simulink model "untitled"  (R2022a)
settings: Solver=FixedStepDiscrete  StartTime=0.0  StopTime=10.0  RelTol=1e-3  EnableMultiTasking=on
model workspace (MATLAB code in the model file):
  | cmdLim = Simulink.Parameter;
  | cmdLim.Value = 15;
  | cmdLim.Description = 'Limit for controlling the maximum surface command angle.';
  | cmdLim.Min = 0;
  | cmdLim.Max = 90;
  | cmdLim.DocUnits = 'deg';
  | 
  | dispGain = Simulink.Parameter;
  | dispGain.Value = 0.75;
  | dispGain.Description = 'Gain applied to the displacement error.';
  | dispGain.Min = 0;
  | dispGain.Max = [];
  | dispGain.DocUnits = 'deg/sec/deg';
  | 
  | dispLim = Simulink.Parameter;
  | dispLim.Value = 30;
  | dispLim.Description = 'Limit for controlling the maximum commanded angle.';
  | dispLim.Min = 0;
  | dispLim.Max = 180;
  | dispLim.DocUnits = 'deg';
  | 
  | intGain = Simulink.Parameter;
  | intGain.Value = 0.5;
  | intGain.Description = 'Gain applied to the integral error.';
  | intGain.Min = 0;
  | intGain.Max = [];
  | intGain.DocUnits = 'deg/sec/deg/sec';
  | 
  | intLim = Simulink.Parameter;
  | intLim.Value = 5;
  | intLim.Description = 'Limit for controlling the maximum commanded angle.';
  | intLim.Min = 0;
  | intLim.Max = 90;
  | intLim.DocUnits = 'deg';
  | 
  | rateGain = Simulink.Parameter;
  | rateGain.Value = 2;
  | rateGain.Description = 'Gain applied to the rate error.';
  | rateGain.Min = 0;
  | rateGain.Max = [];
  | rateGain.DocUnits = 'deg/deg/sec';
  | 
  | rateLim = Simulink.Parameter;
  | rateLim.Value = 6;
  | rateLim.Description = 'Limit for controlling the maximum commanded angle.';
  | rateLim.Min = 0;
  | rateLim.Max = 180;
  | rateLim.DocUnits = 'deg/sec';
  | 
  | hdgGain = Simulink.Parameter;
  | hdgGain.Value = 0.015;
settings Model: RequirementInfo={} %GIDa_fe9045fd_0412_4b6e_8206_617cc20e6fde  FPTRunName=Active  FPTShortcutValueString='{{},{''BaselineRun'',1,1,1,''BaselineRun'','''',{},''M'','''',''''},{''EmbeddedRun'',1,1,1,''EmbeddedRun'','''',{},''M'','''',''''}}'  ExtModeTrigDuration=2  Creator=Amin  LastModifiedBy=Amin
settings SolverCC: AlgebraicLoopSolver=TrustRegion  AutoInsertRateTranBlk=on  MaxZcPerStep=1
settings DataIOCC: SaveOutput=off  SignalLogging=off  DSMLogging=off  SaveTime=off
settings OptimizationCC: UseDivisionForNetSlopeComputation=on  GainParamInheritBuiltInType=on  UseFloatMulNetSlope=on  UseSpecifiedMinMax=on  EnhancedBackFolding=on  PassReuseOutputArgsAs=Individual arguments  ZeroExternalMemoryAtStartup=off  ZeroInternalMemoryAtStartup=off  NoFixptDivByZeroProtection=on  EfficientFloat2IntCast=on  LifeSpan=1  MaxStackSize=64  OptimizeBlockOrder=speed  DifferentSizesBufferReuse=on  OptimizationCustomize=off  EfficientTunableParamExpr=on
settings DebuggingCC: SignalRangeChecking=warning  AllowSymbolicDim=off  SFUnexpectedBacktrackingDiag=warning  SFNoUnconditionalDefaultTransitionDiag=warning  SFExecutionAtInitializationDiag=none  ArithmeticOperatorsInVariantConditions=warning
settings HardwareCC: ProdBitPerInt=16  ProdBitPerPointer=16  ProdBitPerSizeT=16  ProdBitPerPtrDiffT=16  ProdLargestAtomicFloat=None  ProdWordSize=8  ProdHWDeviceType=Atmel->AVR
settings SFSimCC: MATLABDynamicMemAlloc=off
settings RTWCC: SystemTargetFile=ert.tlc  HardwareBoard=Arduino Mega 2560  TemplateMakefile=ert_default_tmf  Toolchain=Arduino AVR  BuildConfiguration=Faster Runs
settings CodeAppCC: ForceParamTrailComments=on  IgnoreCustomStorageClasses=off  OperatorAnnotations=on  SimulinkDataObjDesc=on  SFDataObjDesc=on  CustomSymbolStrGlobalVar=rt$N$M  CustomSymbolStrType=$N$M  CustomSymbolStrFcn=$N$M$F  CustomSymbolStrMacro=$N$M  InsertBlockDesc=on  EnableCustomComments=on  ReqsInCode=on
settings ERTTargetCC: UtilityFuncGeneration=Shared location  MultiwordLength=2048  IncludeMdlTerminateFcn=off  CombineSignalStateStructs=on  SuppressErrorStatus=on  SupportAbsoluteTime=off  SupportNonFinite=off  SupportComplex=off  SupportContinuousTime=on  SupportVariableSizeSignals=on  ExtModeTransport=3  ExtModeStaticAlloc=on  ExtModeStaticAllocSize=2048  ExtModeMexFile=ext_xcp  ExtModeIntrfLevel=Level2 - Open  ERTFilePackagingFormat=CompactWithDataFile
settings ConfigComp: CovScope=ReferencedModels  CovSaveName=covdata_rollAP  CovMetricSettings=dcmtrwe  CovHTMLOptions=-sRT=1 -aTS=1 -bRG=1 -bTC=1 -hTR=1 -nFC=0 -scm=1 -bcm=1 -xEv=0  CovSaveCumulativeToWorkspaceVar=on  CovSaveSingleToWorkspaceVar=on  CovCumulativeVarName=covCumulativeData_rollAP  CovReportOnPause=off  CovExternalEMLEnable=off  CovSFcnEnable=off

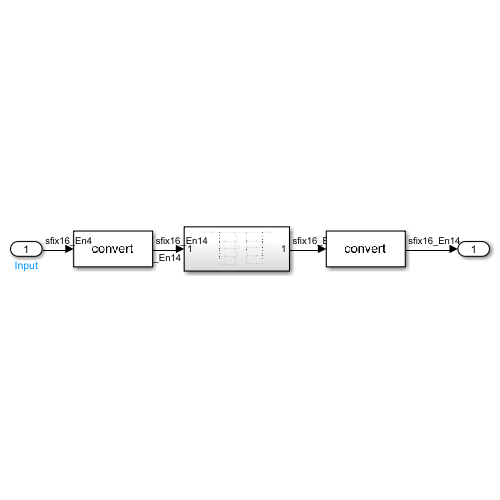
[thumbnail: Simulink's stored preview of the top-level diagram]
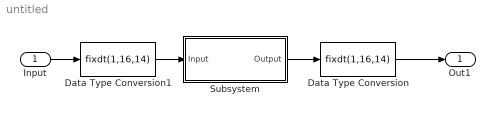
== system untitled ==
  Input : Inport  OutDataTypeStr=fixdt(1,16,4)
  Data Type Conversion : DataTypeConversion  OutDataTypeStr=fixdt(1,16,14)  SaturateOnIntegerOverflow=off  RndMeth=Floor
  Data Type Conversion1 : DataTypeConversion  OutDataTypeStr=fixdt(1,16,14)  SaturateOnIntegerOverflow=off  RndMeth=Floor
  Subsystem : Subsystem
  Out1 : Outport
  wires:
  Data Type Conversion1/1 -> Subsystem/1(Input)
  Input/1 -> Data Type Conversion1/1
  Data Type Conversion/1 -> Out1/1
  Subsystem/1(Output) -> Data Type Conversion/1

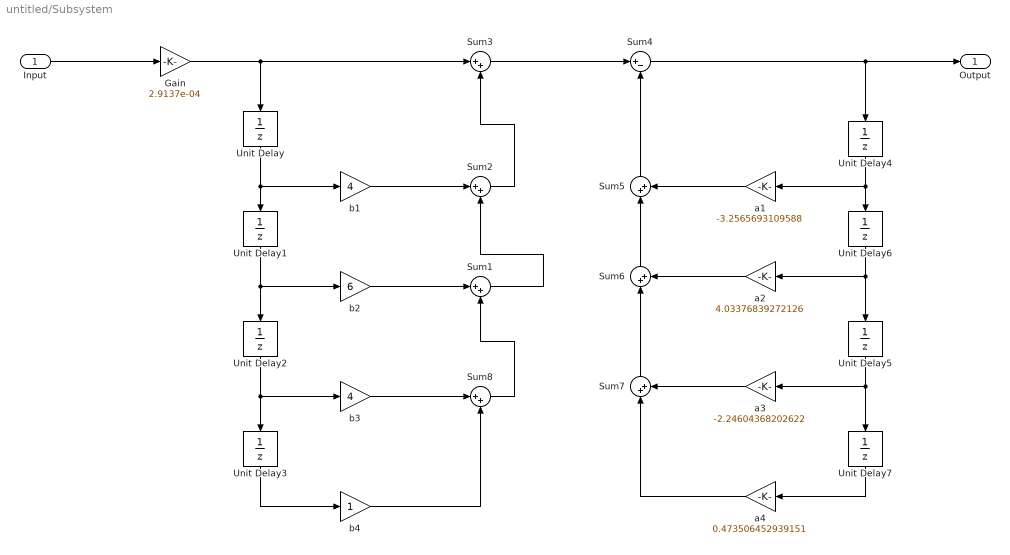
== system untitled/Subsystem ==
  Input : Inport  OutDataTypeStr=fixdt(1,16,14)
  Gain : Gain  Gain=2.9137e-04  OutDataTypeStr=fixdt(1,16,26)
  Sum1 : Sum  Inputs=|++  OutDataTypeStr=fixdt(1,16,23)
  Sum2 : Sum  Inputs=|++  OutDataTypeStr=fixdt(1,16,22)
  Sum3 : Sum  Inputs=|++  OutDataTypeStr=fixdt(1,16,22)
  Sum4 : Sum  Inputs=|+-  OutDataTypeStr=fixdt(1,16,14)
  Sum5 : Sum  Inputs=|++  OutDataTypeStr=fixdt(1,16,14)
  Sum6 : Sum  Inputs=|++  OutDataTypeStr=fixdt(1,16,13)
  Sum7 : Sum  Inputs=|++  OutDataTypeStr=fixdt(1,16,14)
  Sum8 : Sum  Inputs=|++  OutDataTypeStr=fixdt(1,16,24)
  Unit Delay{,1..7} (8 alike) : UnitDelay  SampleTime=-1  HasFrameUpgradeWarning=on
  a1 : Gain  Gain=-3.2565693109588  OutDataTypeStr=fixdt(1,16,13)
  a2 : Gain  Gain=4.03376839272126  OutDataTypeStr=fixdt(1,16,12)
  a3 : Gain  Gain=-2.24604368202622  OutDataTypeStr=fixdt(1,16,13)
  a4 : Gain  Gain=0.473506452939151  OutDataTypeStr=fixdt(1,16,16)
  b1 : Gain  Gain=4  OutDataTypeStr=fixdt(1,16,24)
  b2 : Gain  Gain=6  OutDataTypeStr=fixdt(1,16,23)
  b3 : Gain  Gain=4  OutDataTypeStr=fixdt(1,16,24)
  b4 : Gain  OutDataTypeStr=fixdt(1,16,26)
  Output : Outport
  wires:
  b3/1 -> Sum8/1
  Unit Delay4/1 -> Unit Delay6/1, a1/1
  Input/1 -> Gain/1
  Sum4/1 -> Output/1, Unit Delay4/1
  Unit Delay/1 -> b1/1, Unit Delay1/1
  Unit Delay3/1 -> b4/1
  Sum1/1 -> Sum2/2
  a4/1 -> Sum7/1
  a1/1 -> Sum5/2
  a3/1 -> Sum7/2
  Sum8/1 -> Sum1/2
  Unit Delay6/1 -> a2/1, Unit Delay5/1
  b1/1 -> Sum2/1
  Sum5/1 -> Sum4/2
  Unit Delay5/1 -> a3/1, Unit Delay7/1
  a2/1 -> Sum6/2
  b4/1 -> Sum8/2
  b2/1 -> Sum1/1
  Unit Delay2/1 -> b3/1, Unit Delay3/1
  Sum7/1 -> Sum6/1
  Gain/1 -> Sum3/1, Unit Delay/1
  Sum2/1 -> Sum3/2
  Unit Delay1/1 -> b2/1, Unit Delay2/1
  Unit Delay7/1 -> a4/1
  Sum3/1 -> Sum4/1
  Sum6/1 -> Sum5/1
